simulink model "Radar_V1_1"  (R2018a)
settings: Solver=VariableStepAuto  StartTime=0.0  StopTime=10.0  FixedStep=sampletime  RelTol=1e-3  EnableMultiTasking=on
PreLoadFcn:
  | Radar_V1_BusInfo;
libraries: simulink x2
settings Model: Creator=IAEC nishito  LastModifiedBy=nishito
settings DataIOCC: LimitDataPoints=on  SaveFormat=Array  SignalLoggingSaveFormat=ModelDataLogs  SaveOutput=off
settings OptimizationCC: DefaultParameterBehavior=Inlined  ExpressionDepthLimit=2147483647  LifeSpan=inf
settings DebuggingCC: UnderspecifiedInitializationDetection=Classic  MergeDetectMultiDrivingBlocksExec=none  SolverPrmCheckMsg=warning  FcnCallInpInsideContextMsg=warning  StateNameClashWarn=warning  SFUnexpectedBacktrackingDiag=warning  SFNoUnconditionalDefaultTransitionDiag=warning  SFExecutionAtInitializationDiag=none
settings HardwareCC: ProdBitPerPointer=32  ProdBitPerSizeT=32  ProdBitPerPtrDiffT=32  ProdLargestAtomicFloat=None  ProdIntDivRoundTo=Undefined  ProdEndianess=Unspecified  ProdWordSize=32  ProdHWDeviceType=32-bit Generic
settings ModelReferenceCC: UpdateModelReferenceTargets=IfOutOfDate  PropagateSignalLabelsOutOfModel=off
settings CodeAppCC: StateflowObjectComments=on
settings GRTTargetCC: TargetLangStandard=C89/C90 (ANSI)  GeneratePreprocessorConditionals=Disable all  CombineOutputUpdateFcns=off  GRTInterface=on
settings ConfigComp: CovMetricSettings=dw  CovHtmlReporting=on  CovSaveCumulativeToWorkspaceVar=on  CovSaveSingleToWorkspaceVar=on  CovExternalEMLEnable=off

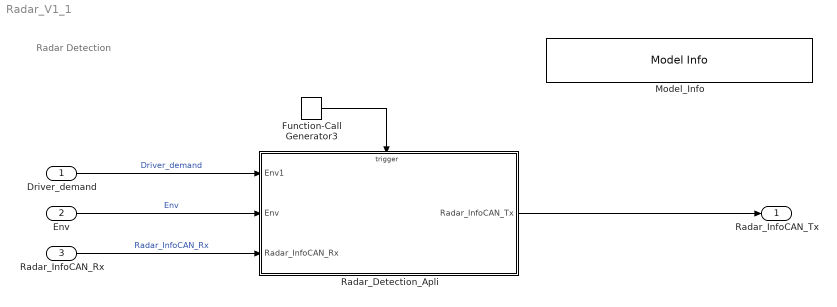
== system Radar_V1_1 ==
  note: Radar Detection
  Driver_demand : Inport  OutDataTypeStr=Bus: Driver_demand_Bus
      settings: AttributesFormatString=<%<OutDataTypeStr>>
  Env : Inport  Port=2  OutDataTypeStr=Bus: Environment_Bus
      settings: AttributesFormatString=<%<OutDataTypeStr>>
  Radar_InfoCAN_Rx : Inport  Port=3  OutDataTypeStr=Bus: Radar_InfoCAN_Rx_Bus
      settings: AttributesFormatString=<%<OutDataTypeStr>>
  Function-Call Generator3 : simulink/Ports & Subsystems/Function-Call Generator  sample_time=0.1  numberOfIterations=1
      settings: AttributesFormatString=<sample_time=%<sample_time>>
  Model_Info : simulink/Model-Wide Utilities/Model Info  Frame=on  DisplayStringWithTags=|  HorizontalTextAlignment=Left  LeftAlignmentValue=0.02
      | Version  %<ModelVersion>
      | LastModifided by %<LastModifiedBy>  Date %<LastModificationDate>
      | Description  %<Description>
  Radar_Detection_Apli : Subsystem
  Radar_InfoCAN_Tx : Outport  OutDataTypeStr=Bus: Radar_InfoCAN_Tx_Bus
      settings: AttributesFormatString=<%<OutDataTypeStr>>
  wires:
  Radar_Detection_Apli/1(Radar_InfoCAN_Tx) -> Radar_InfoCAN_Tx/1
  Radar_InfoCAN_Rx/1 -> Radar_Detection_Apli/3(Radar_InfoCAN_Rx)  "Radar_InfoCAN_Rx"
  Env/1 -> Radar_Detection_Apli/2(Env)  "Env"
  Function-Call Generator3/1 -> Radar_Detection_Apli/Trigger
  Driver_demand/1 -> Radar_Detection_Apli/1(Env1)  "Driver_demand"

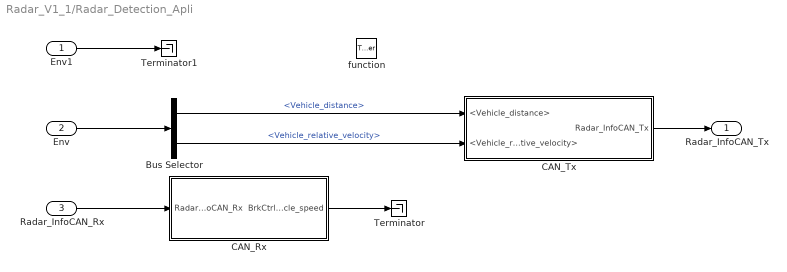
== system Radar_V1_1/Radar_Detection_Apli ==
  Env1 : Inport
  Env : Inport  Port=2
  Radar_InfoCAN_Rx : Inport  Port=3
  function : TriggerPort  TriggerType=function-call  VariantControl=Variant
  Bus Selector : BusSelector  OutputSignals=Vehicle_distance,Vehicle_relative_velocity
  CAN_Rx : Subsystem
  CAN_Tx : Subsystem
  Terminator : Terminator
  Terminator1 : Terminator
  Radar_InfoCAN_Tx : Outport
  wires:
  Env/1 -> Bus Selector/1
  Bus Selector/1 -> CAN_Tx/1(<Vehicle_distance>)  "<Vehicle_distance>"
  Bus Selector/2 -> CAN_Tx/2(<Vehicle_relative_velocity>)  "<Vehicle_relative_velocity>"
  CAN_Tx/1(Radar_InfoCAN_Tx) -> Radar_InfoCAN_Tx/1
  Radar_InfoCAN_Rx/1 -> CAN_Rx/1(Radar_InfoCAN_Rx)
  CAN_Rx/1(BrkCtrl_Vehicle_speed) -> Terminator/1
  Env1/1 -> Terminator1/1

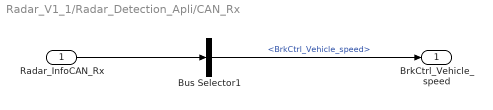
== system Radar_V1_1/Radar_Detection_Apli/CAN_Rx ==
  Radar_InfoCAN_Rx : Inport
  Bus Selector1 : BusSelector  OutputSignals=BrkCtrl_Vehicle_speed
  BrkCtrl_Vehicle_speed : Outport
  wires:
  Radar_InfoCAN_Rx/1 -> Bus Selector1/1
  Bus Selector1/1 -> BrkCtrl_Vehicle_speed/1  "<BrkCtrl_Vehicle_speed>"

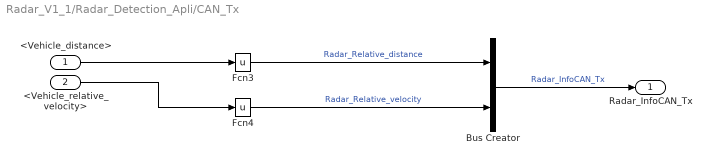
== system Radar_V1_1/Radar_Detection_Apli/CAN_Tx ==
  <Vehicle_distance> : Inport
  <Vehicle_relative_velocity> : Inport  Port=2
  Bus Creator : BusCreator  Inputs=2  OutDataTypeStr=Bus: Radar_InfoCAN_Tx_Bus
      settings: AttributesFormatString=<%<OutDataTypeStr>>
  Fcn3 : Fcn  Expr=u
  Fcn4 : Fcn  Expr=u
  Radar_InfoCAN_Tx : Outport
  wires:
  Fcn4/1 -> Bus Creator/2  "Radar_Relative_velocity"
  Fcn3/1 -> Bus Creator/1  "Radar_Relative_distance"
  Bus Creator/1 -> Radar_InfoCAN_Tx/1  "Radar_InfoCAN_Tx"
  <Vehicle_distance>/1 -> Fcn3/1
  <Vehicle_relative_velocity>/1 -> Fcn4/1
